simulink model "PubIfCommonEHRV2_MDL"  (R2020b)
settings: Solver=FixedStepAuto  StartTime=0.0  StopTime=Inf  RelTol=1e-3
PostLoadFcn:
  | if any(exist('dsrtsu_mdlpostloadfcn', 'file') ~= 0), dsrtsu_mdlpostloadfcn('Execute', bdroot); end
InitFcn:
  | , if any(exist('dsmpb_private', 'file') ~= 0), dsmpb_private('dsmpb_mdlclblib', 'Init', bdroot); end,
undefined symbols (not defined in the file): CAMERA_STATE_INITIAL, CAMERA_STATE_NORMAL, CURVATURE_UNKNOWN, DISTANCE_UNKONWN, DRIVING_ON_HIGHWAY_YES, EHR_CYCLE, FORWARD_LOOKING_DISTANCE_LIMIT, IFC_HUT_INTERFACE_NO_RESPONSE, IFC_HUT_INTERFACE_RESPONSE, MAP_DATA_VALID_VALID, MSG_TYPE_PROFILE_LONG, MSG_TYPE_PROFILE_SHORT, MSG_TYPE_SEGMENT, MSG_TYPE_STUB, OFFSET_INVALID, OFFSET_MAX, P_EHRV2_dCurvatureFar, P_EHRV2_dCurvatureMatrix, P_EHRV2_dSlopeFar, P_EHRV2_dSlopeMatrix, P_EHRV2_dVehForwardLooking, P_EHRV2_dVehRearLooking, P_EHRV2_tIFCHUTNoResponseOfForecastTreeReset, P_EHRV2_tIFCHUTNoResponseOfTimeout, P_EHRV2_tIFCHUTResponseTimeout, PROFILE_SHORT_NO_OTHER_VALUE, PROFILE_SHORT_TYPE_CURVATURE, PROFILE_SHORT_TYPE_SLOPE, REAR_LOOKING_DISTANCE_LIMIT, SLOPE_UNKNOWN, STUB_CMPLX_INSCT, STUB_FORM_OF_WAY_HIGH_RING_ROAD, STUB_FORM_OF_WAY_NORMAL_RING_ROAD
libraries: simulink x5
(part 4 of 4)

== matlab function PubIfCommonEHRV2_MDL/EHR/EHR_Main/DS_Calc_ProfileShortIsInDataWindow ==
  data: PositionStruct input; ProfileShortIsInDataWindow output boolean; ProfileShortStruct input; StubVector input; StubVectorSize input; P_EHRV2_dVehRearLooking parameter; P_EHRV2_dVehForwardLooking parameter
function ProfileShortIsInDataWindow = fcn(PositionStruct, ProfileShortStruct,...
    StubVector, StubVectorSize,...
    P_EHRV2_dVehRearLooking, P_EHRV2_dVehForwardLooking)

t_flag = false;  %Whether the valid stub data can be found

%%%%%%%%%Position Road%%%%%%%%%
if ProfileShortStruct.ProfShortPathIdx == PositionStruct.PosnPathIdx
    if (ProfileShortStruct.ProfShortRelativeOffset >= P_EHRV2_dVehRearLooking)...
        && (ProfileShortStruct.ProfShortRelativeOffset <= P_EHRV2_dVehForwardLooking)
        ProfileShortIsInDataWindow = true;
    else
        ProfileShortIsInDataWindow = false;
    end
%%%%%%%%%Other Road%%%%%%%%%
else
    %%%%iterator overflow prevention%%%%
    if 0 == StubVectorSize
        ProfileShortIsInDataWindow = false;
    else
       for t = 1:StubVectorSize
           if ProfileShortStruct.ProfShortPathIdx == StubVector(t).StubStubPathIdx
               t_flag = true;
               break;
           end
       end
       if true == t_flag   %This is stub
           ProfileShortIsInDataWindow = true;
       else
           ProfileShortIsInDataWindow = false;
       end
    end
end

== matlab function PubIfCommonEHRV2_MDL/EHR/EHR_Main/DS_Calc_ProfileShortIsUpdated ==
  data: ProfileShortStruct input; ProfileShortIsUpdated output boolean; ProfileShortVector input; ProfileShortVectorSize input
function ProfileShortIsUpdated = fcn(ProfileShortStruct, ProfileShortVector, ProfileShortVectorSize)

if 0 == ProfileShortStruct.ProfShortMsgType   %Means this struct is null
    ProfileShortIsUpdated = false;
else
    %%%%overflow prevention%%%%
    if 0 == ProfileShortVectorSize
        ProfileShortIsUpdated = true;
    elseif (ProfileShortStruct.ProfShortOffset == ProfileShortVector(ProfileShortVectorSize).ProfShortOffset)...
             && (ProfileShortStruct.ProfShortCycCnt == ProfileShortVector(ProfileShortVectorSize).ProfShortCycCnt)
        ProfileShortIsUpdated = false;
    else
        ProfileShortIsUpdated = true;
    end
end

== matlab function PubIfCommonEHRV2_MDL/EHR/EHR_Main/DS_Calc_ProfileShortVector ==
  data: PositionStruct input; ProfileShortVector output Bus: ProfileShortStruct size=200; PositionStructK1 input; ProfileShortStruct input; ProfileShortIsUpdated input; ProfileShortIsInDataWindow input; ForecastTreeResetFlag input; StubVector input; StubVectorSize input; ProfileShortVectorK1 input; ProfileShortVectorSizeK1 input; ProfileShortVectorSize output uint16; OFFSET_INVALID parameter; REAR_LOOKING_DISTANCE_LIMIT parameter; FORWARD_LOOKING_DISTANCE_LIMIT parameter; OFFSET_MAX parameter; P_EHRV2_dVehRearLooking parameter; P_EHRV2_dVehForwardLooking parameter
function [ProfileShortVector, ProfileShortVectorSize] = fcn(PositionStruct, PositionStructK1, ProfileShortStruct,...
    ProfileShortIsUpdated, ProfileShortIsInDataWindow, ForecastTreeResetFlag,...
    StubVector, StubVectorSize, ProfileShortVectorK1, ProfileShortVectorSizeK1,...
    OFFSET_INVALID, REAR_LOOKING_DISTANCE_LIMIT, FORWARD_LOOKING_DISTANCE_LIMIT, OFFSET_MAX, P_EHRV2_dVehRearLooking, P_EHRV2_dVehForwardLooking)

ProfileShortVector = ProfileShortVectorK1;
ProfileShortVectorSize = ProfileShortVectorSizeK1;

if true == ForecastTreeResetFlag
    for t = 1:ProfileShortVectorSize
        ProfileShortVector(t).ProfShortOffset = uint16(0);
        ProfileShortVector(t).ProfShortMsgType = uint8(0);
        ProfileShortVector(t).ProfShortPathIdx = uint8(0);
        ProfileShortVector(t).ProfShortCycCnt = uint8(0);
        ProfileShortVector(t).ProfShortUpdate = false;
        ProfileShortVector(t).ProfShortRetr = false;
        ProfileShortVector(t).ProfShortCtrlPoint = false;
        ProfileShortVector(t).ProfShortProfType = uint8(0);
        ProfileShortVector(t).ProfShortDist1 = uint16(0);
        ProfileShortVector(t).ProfShortAccurClass = uint8(0);
        ProfileShortVector(t).ProfShortValue0 = uint16(0);
        ProfileShortVector(t).ProfShortValue1 = uint16(0);
        ProfileShortVector(t).ProfShortRelativeOffset = int16(0);
    end
    ProfileShortVectorSize = uint16(0);
else
    %%%%%Update Actual Offset AND Delete%%%%%
    if (false == isequal(PositionStruct,PositionStructK1)) && (PositionStruct.PosnPathIdx > 3)   %Position is updated
        ProfileShortVectorSize = uint16(0);   %ProfileShortVectorSize need to be calculated again
        %%%%overflow prevention%%%%
        if 0 == ProfileShortVectorSizeK1
            %Do nothing
        else
            for t = 1:ProfileShortVectorSizeK1
                %%%%%Update Actual Offset%%%%%
                ProfileShortVector(t).ProfShortRelativeOffset = EHR_Calc_RelativeOffset(PositionStruct,ProfileShortVector(t).ProfShortPathIdx,ProfileShortVector(t).ProfShortOffset);
                %%%%%Delete%%%%%
                if DS_Calc_ProfileShortNeedDelete(PositionStruct,ProfileShortVector(t),P_EHRV2_dVehRearLooking,P_EHRV2_dVehForwardLooking,StubVector,StubVectorSize) == true
                    %Do nothing
                else
                    ProfileShortVectorSize = ProfileShortVectorSize + 1;
                    ProfileShortVector(ProfileShortVectorSize) = ProfileShortVector(t);
                end
            end
        end
    else
        %Do nothing
    end

    %%%%%Store%%%%%
    if (true == ProfileShortIsUpdated) && (true == ProfileShortIsInDataWindow) && (ProfileShortStruct.ProfShortPathIdx > 7)
        ProfileShortVectorSize = ProfileShortVectorSize + 1;
        if ProfileShortVectorSize <= length(ProfileShortVector)
            ProfileShortVector(ProfileShortVectorSize) = ProfileShortStruct;
        else
            ProfileShortVectorSize = uint16(length(ProfileShortVector));
        end
    else
        %Do nothing
    end

    if ProfileShortVectorSize < ProfileShortVectorSizeK1
        for t = (ProfileShortVectorSize + 1):ProfileShortVectorSizeK1
            ProfileShortVector(t).ProfShortOffset = uint16(0);
            ProfileShortVector(t).ProfShortMsgType = uint8(0);
            ProfileShortVector(t).ProfShortPathIdx = uint8(0);
            ProfileShortVector(t).ProfShortCycCnt = uint8(0);
            ProfileShortVector(t).ProfShortUpdate = false;
            ProfileShortVector(t).ProfShortRetr = false;
            ProfileShortVector(t).ProfShortCtrlPoint = false;
            ProfileShortVector(t).ProfShortProfType = uint8(0);
            ProfileShortVector(t).ProfShortDist1 = uint16(0);
            ProfileShortVector(t).ProfShortAccurClass = uint8(0);
            ProfileShortVector(t).ProfShortValue0 = uint16(0);
            ProfileShortVector(t).ProfShortValue1 = uint16(0);
            ProfileShortVector(t).ProfShortRelativeOffset = int16(0);
        end
    end
end

== matlab function PubIfCommonEHRV2_MDL/EHR/EHR_Main/DS_Calc_SegmentIsInDataWindow ==
  data: PositionStruct input; SegmentIsInDataWindow output boolean; SegmentStruct input; StubVector input; StubVectorSize input; P_EHRV2_dVehRearLooking parameter; P_EHRV2_dVehForwardLooking parameter
function SegmentIsInDataWindow = fcn(PositionStruct, SegmentStruct,...
    StubVector, StubVectorSize,...
    P_EHRV2_dVehRearLooking, P_EHRV2_dVehForwardLooking)

t_flag = false;  %Whether the valid stub data can be found

%%%%%%%%%Position Road%%%%%%%%%
if SegmentStruct.SegPathIdx == PositionStruct.PosnPathIdx
    if (SegmentStruct.SegRelativeOffset >= P_EHRV2_dVehRearLooking)...
        && (SegmentStruct.SegRelativeOffset <= P_EHRV2_dVehForwardLooking)
        SegmentIsInDataWindow = true;
    else
        SegmentIsInDataWindow = false;
    end
%%%%%%%%%Other Road%%%%%%%%%
else
    %%%%iterator overflow prevention%%%%
    if 0 == StubVectorSize
        SegmentIsInDataWindow = false;
    else
       for t = 1:StubVectorSize
           if SegmentStruct.SegPathIdx == StubVector(t).StubStubPathIdx
               t_flag = true;
               break;
           end
       end
       if true == t_flag   %This is stub
           SegmentIsInDataWindow = true;
       else
           SegmentIsInDataWindow = false;
       end
    end
end

== matlab function PubIfCommonEHRV2_MDL/EHR/EHR_Main/DS_Calc_SegmentIsUpdated ==
  data: SegmentStruct input; SegmentIsUpdated output boolean; SegmentVector input; SegmentVectorSize input
function SegmentIsUpdated = fcn(SegmentStruct, SegmentVector, SegmentVectorSize)

if 0 == SegmentStruct.SegMsgType   %Means this struct is null
    SegmentIsUpdated = false;
else
    %%%%overflow prevention%%%%
    if 0 == SegmentVectorSize
        SegmentIsUpdated = true;
    elseif (SegmentStruct.SegOffset == SegmentVector(SegmentVectorSize).SegOffset)...
             && (SegmentStruct.SegCycCnt == SegmentVector(SegmentVectorSize).SegCycCnt)
        SegmentIsUpdated = false;
    else
        SegmentIsUpdated = true;
    end
end

== matlab function PubIfCommonEHRV2_MDL/EHR/EHR_Main/DS_Calc_SegmentVector ==
  data: PositionStruct input; SegmentVector output Bus: SegmentStruct size=400; PositionStructK1 input; SegmentStruct input; SegmentIsUpdated input; SegmentIsInDataWindow input; ForecastTreeResetFlag input; StubVector input; StubVectorSize input; SegmentVectorK1 input; SegmentVectorSizeK1 input; SegmentVectorSize output uint16; OFFSET_INVALID parameter; REAR_LOOKING_DISTANCE_LIMIT parameter; FORWARD_LOOKING_DISTANCE_LIMIT parameter; OFFSET_MAX parameter; P_EHRV2_dVehRearLooking parameter; P_EHRV2_dVehForwardLooking parameter
function [SegmentVector, SegmentVectorSize] = fcn(PositionStruct, PositionStructK1, SegmentStruct,...
    SegmentIsUpdated, SegmentIsInDataWindow, ForecastTreeResetFlag,...
    StubVector, StubVectorSize, SegmentVectorK1, SegmentVectorSizeK1,...
    OFFSET_INVALID, REAR_LOOKING_DISTANCE_LIMIT, FORWARD_LOOKING_DISTANCE_LIMIT, OFFSET_MAX, P_EHRV2_dVehRearLooking, P_EHRV2_dVehForwardLooking)

SegmentVector = SegmentVectorK1;
SegmentVectorSize = SegmentVectorSizeK1;

if true == ForecastTreeResetFlag
    for t = 1:SegmentVectorSize
        SegmentVector(t).SegOffset = uint16(0);
        SegmentVector(t).SegMsgType = uint8(0);
        SegmentVector(t).SegPathIdx = uint8(0);
        SegmentVector(t).SegCycCnt = uint8(0);
        SegmentVector(t).SegUpdate = false;
        SegmentVector(t).SegRetr = false;
        SegmentVector(t).SegBuildUpArea = uint8(0);
        SegmentVector(t).SegBridge = uint8(0);
        SegmentVector(t).SegTunnel = uint8(0);
        SegmentVector(t).SegFuncRoadClass = uint8(0);
        SegmentVector(t).SegRelProbb = single(0);
        SegmentVector(t).SegFormOfWay = uint8(0);
        SegmentVector(t).SegCmplxInsct = uint8(0);
        SegmentVector(t).SegPartOfCalcRoute = uint8(0);
        SegmentVector(t).SegEffSpdLmtType = uint8(0);
        SegmentVector(t).SegEffSpdLmt = uint8(0);
        SegmentVector(t).SegNumOfLaneDrvDir = uint8(0);
        SegmentVector(t).SegNumOfLaneOppDir = uint8(0);
        SegmentVector(t).SegDivideRoad = uint8(0);
        SegmentVector(t).SegRelativeOffset = int16(0);
    end
    SegmentVectorSize = uint16(0);
else
    %%%%%Update Actual Offset AND Delete%%%%%
    if (false == isequal(PositionStruct,PositionStructK1)) && (PositionStruct.PosnPathIdx > 3)   %Position is updated
        SegmentVectorSize = uint16(0);   %SegmentVectorSize need to be calculated again
        %%%%overflow prevention%%%%
        if 0 == SegmentVectorSizeK1
            %Do nothing
        else
            for t = 1:SegmentVectorSizeK1
                %%%%%Update Actual Offset%%%%%
                SegmentVector(t).SegRelativeOffset = EHR_Calc_RelativeOffset(PositionStruct,SegmentVector(t).SegPathIdx,SegmentVector(t).SegOffset);
                %%%%%Delete%%%%%
                if DS_Calc_SegmentNeedDelete(PositionStruct,SegmentVector(t),P_EHRV2_dVehRearLooking,P_EHRV2_dVehForwardLooking,StubVector,StubVectorSize) == true
                    %Do nothing
                else
                    SegmentVectorSize = SegmentVectorSize + 1;
                    SegmentVector(SegmentVectorSize) = SegmentVector(t);
                end
            end
        end
    else
        %Do nothing
    end

    %%%%%Store%%%%%
    if (true == SegmentIsUpdated) && (true == SegmentIsInDataWindow) && (SegmentStruct.SegPathIdx > 7)
        SegmentVectorSize = SegmentVectorSize + 1;
        if SegmentVectorSize <= length(SegmentVector)
            SegmentVector(SegmentVectorSize) = SegmentStruct;
        else
            SegmentVectorSize = uint16(length(SegmentVector));
        end
    else
        %Do nothing
    end

    if SegmentVectorSize < SegmentVectorSizeK1
        for t = (SegmentVectorSize + 1):SegmentVectorSizeK1
            SegmentVector(t).SegOffset = uint16(0);
            SegmentVector(t).SegMsgType = uint8(0);
            SegmentVector(t).SegPathIdx = uint8(0);
            SegmentVector(t).SegCycCnt = uint8(0);
            SegmentVector(t).SegUpdate = false;
            SegmentVector(t).SegRetr = false;
            SegmentVector(t).SegBuildUpArea = uint8(0);
            SegmentVector(t).SegBridge = uint8(0);
            SegmentVector(t).SegTunnel = uint8(0);
            SegmentVector(t).SegFuncRoadClass = uint8(0);
            SegmentVector(t).SegRelProbb = single(0);
            SegmentVector(t).SegFormOfWay = uint8(0);
            SegmentVector(t).SegCmplxInsct = uint8(0);
            SegmentVector(t).SegPartOfCalcRoute = uint8(0);
            SegmentVector(t).SegEffSpdLmtType = uint8(0);
            SegmentVector(t).SegEffSpdLmt = uint8(0);
            SegmentVector(t).SegNumOfLaneDrvDir = uint8(0);
            SegmentVector(t).SegNumOfLaneOppDir = uint8(0);
            SegmentVector(t).SegDivideRoad = uint8(0);
            SegmentVector(t).SegRelativeOffset = int16(0);
        end
    end
end

== matlab function PubIfCommonEHRV2_MDL/EHR/EHR_Main/DS_Calc_StubIsInDataWindow ==
  data: PositionStruct input; StubIsInDataWindow output boolean; StubStruct input; P_EHRV2_dVehRearLooking parameter; P_EHRV2_dVehForwardLooking parameter
function StubIsInDataWindow = fcn(PositionStruct, StubStruct, P_EHRV2_dVehRearLooking, P_EHRV2_dVehForwardLooking)

if (StubStruct.StubPathIdx == PositionStruct.PosnPathIdx)... %Only store 1st level stub
    && (StubStruct.StubRelativeOffset >= P_EHRV2_dVehRearLooking)...
    && (StubStruct.StubRelativeOffset <= P_EHRV2_dVehForwardLooking)
    StubIsInDataWindow = true;
else
    StubIsInDataWindow = false;
end

== matlab function PubIfCommonEHRV2_MDL/EHR/EHR_Main/DS_Calc_StubIsUpdated ==
  data: StubStruct input; StubIsUpdated output boolean; StubVector input; StubVectorSize input
function StubIsUpdated = fcn(StubStruct, StubVector, StubVectorSize)

if 0 == StubStruct.StubMsgType   %Means this struct is null
    StubIsUpdated = false;
else
    %%%%overflow prevention%%%%
    if 0 == StubVectorSize
        StubIsUpdated = true;
    elseif (StubStruct.StubStubPathIdx == StubVector(StubVectorSize).StubStubPathIdx)...
             && (StubStruct.StubCycCnt == StubVector(StubVectorSize).StubCycCnt)
        StubIsUpdated = false;
    else
        StubIsUpdated = true;
    end
end

== matlab function PubIfCommonEHRV2_MDL/EHR/EHR_Main/DS_Calc_StubVector ==
  data: PositionStruct input; StubVector output Bus: StubStruct size=50; PositionStructK1 input; StubStruct input; StubIsUpdated input; StubIsInDataWindow input; ForecastTreeResetFlag input; StubVectorK1 input; StubVectorSizeK1 input; StubVectorSize output uint16; OFFSET_INVALID parameter; REAR_LOOKING_DISTANCE_LIMIT parameter; FORWARD_LOOKING_DISTANCE_LIMIT parameter; OFFSET_MAX parameter; P_EHRV2_dVehRearLooking parameter; P_EHRV2_dVehForwardLooking parameter
function [StubVector, StubVectorSize] = fcn(PositionStruct, PositionStructK1, StubStruct,...
    StubIsUpdated, StubIsInDataWindow, ForecastTreeResetFlag,...
    StubVectorK1, StubVectorSizeK1,...
    OFFSET_INVALID, REAR_LOOKING_DISTANCE_LIMIT, FORWARD_LOOKING_DISTANCE_LIMIT, OFFSET_MAX, P_EHRV2_dVehRearLooking, P_EHRV2_dVehForwardLooking)

StubVector = StubVectorK1;
StubVectorSize = StubVectorSizeK1;

if true == ForecastTreeResetFlag
    for t = 1:StubVectorSize
        StubVector(t).StubOffset = uint16(0);
        StubVector(t).StubMsgType = uint8(0);
        StubVector(t).StubPathIdx = uint8(0);
        StubVector(t).StubCycCnt = uint8(0);
        StubVector(t).StubUpdate = false;
        StubVector(t).StubRetr = false;
        StubVector(t).StubStubPathIdx = uint8(0);
        StubVector(t).StubFuncRoadClass = uint8(0);
        StubVector(t).StubRelProbb = single(0);
        StubVector(t).StubFormOfWay = uint8(0);
        StubVector(t).StubCmplxInsct = uint8(0);
        StubVector(t).StubPartOfCalcRoute = uint8(0);
        StubVector(t).StubTurnAngl = single(0);
        StubVector(t).StubNumOfLaneDrvDir = uint8(0);
        StubVector(t).StubNumOfLaneOppDir = uint8(0);
        StubVector(t).StubRtOfWay = uint8(0);
        StubVector(t).StubLastStub = false;
        StubVector(t).StubRelativeOffset = int16(0);
        StubVector(t).StubTurnAngl = single(0);
    end
    StubVectorSize = uint16(0);
else
    %%%%%Update Actual Offset AND Delete%%%%%
    if (false == isequal(PositionStruct,PositionStructK1)) && (PositionStruct.PosnPathIdx > 3)   %Position is updated
        StubVectorSize = uint16(0);   %StubVectorSize need to be calculated again
        %%%%overflow prevention%%%%
        if 0 == StubVectorSizeK1
            %Do nothing
        else
            for t = 1:StubVectorSizeK1
                %%%%%Update Actual Offset%%%%%
                StubVector(t).StubRelativeOffset = EHR_Calc_RelativeOffset(PositionStruct,StubVector(t).StubPathIdx,StubVector(t).StubOffset);
                %%%%%Delete%%%%%
                if DS_Calc_StubNeedDelete(PositionStruct,StubVector(t),P_EHRV2_dVehRearLooking,P_EHRV2_dVehForwardLooking) == true
                    %Do nothing
                else
                    StubVectorSize = StubVectorSize + 1;
                    StubVector(StubVectorSize) = StubVector(t);
                end
            end
        end
    else
        %Do nothing
    end

    %%%%%Store%%%%%
    if (true == StubIsUpdated) && (true == StubIsInDataWindow) && (StubStruct.StubPathIdx > 7) && (StubStruct.StubStubPathIdx > 7)
        StubVectorSize = StubVectorSize + 1;
        if StubVectorSize <= length(StubVector)
            StubVector(StubVectorSize) = StubStruct;
        else
            StubVectorSize = uint16(length(StubVector));
        end
    else
        %Do nothing
    end

    if StubVectorSize < StubVectorSizeK1
        for t = (StubVectorSize + 1):StubVectorSizeK1
            StubVector(t).StubOffset = uint16(0);
            StubVector(t).StubMsgType = uint8(0);
            StubVector(t).StubPathIdx = uint8(0);
            StubVector(t).StubCycCnt = uint8(0);
            StubVector(t).StubUpdate = false;
            StubVector(t).StubRetr = false;
            StubVector(t).StubStubPathIdx = uint8(0);
            StubVector(t).StubFuncRoadClass = uint8(0);
            StubVector(t).StubRelProbb = single(0);
            StubVector(t).StubFormOfWay = uint8(0);
            StubVector(t).StubCmplxInsct = uint8(0);
            StubVector(t).StubPartOfCalcRoute = uint8(0);
            StubVector(t).StubTurnAngl = single(0);
            StubVector(t).StubNumOfLaneDrvDir = uint8(0);
            StubVector(t).StubNumOfLaneOppDir = uint8(0);
            StubVector(t).StubRtOfWay = uint8(0);
            StubVector(t).StubLastStub = false;
            StubVector(t).StubRelativeOffset = int16(0);
            StubVector(t).StubTurnAngl = single(0);
        end
    end
end

== matlab function PubIfCommonEHRV2_MDL/EHR/EHR_Output/MATLAB Function ==
  data: Matrix input; Matrix1 output; Matrix2 output
function [Matrix1,Matrix2] = fcn(Matrix)

Matrix1 = single(zeros(1,10));
Matrix2 = single(zeros(1,10));
for i = 1 : 10
    Matrix1(i) = Matrix(i,1);
    Matrix2(i) = Matrix(i,2);
end

== matlab function PubIfCommonEHRV2_MDL/EHR/EHR_Output/MATLAB Function1 ==
  data: Matrix input; Matrix1 output; Matrix2 output
function [Matrix1,Matrix2] = fcn(Matrix)

Matrix1 = single(zeros(1,10));
Matrix2 = single(zeros(1,10));
for i = 1 : 10
    Matrix1(i) = Matrix(i,1);
    Matrix2(i) = Matrix(i,2);
end
